simulink library "LIB_TIME"  (Simulink 8.8)
settings: Solver=ode45  StartTime=0.0  StopTime=10.0  RelTol=1e-3  EnableMultiTasking=on
settings Model: Creator=alger  LastModifiedBy=alger

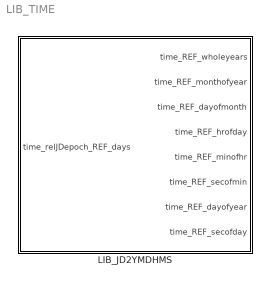
== system LIB_TIME ==
  LIB_JD2YMDHMS : Subsystem  TreatAsAtomicUnit=on

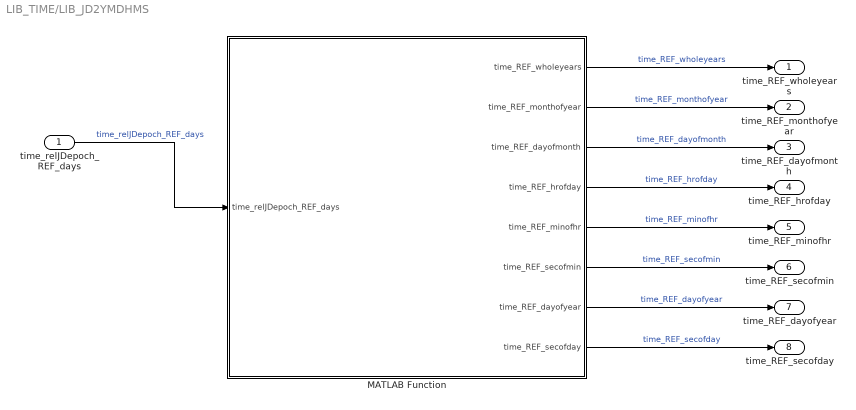
== system LIB_TIME/LIB_JD2YMDHMS ==
  time_relJDepoch_REF_days : Inport
  MATLAB Function : MATLAB Function  TreatAsAtomicUnit=on
  time_REF_wholeyears : Outport
  time_REF_monthofyear : Outport  Port=2
  time_REF_dayofmonth : Outport  Port=3
  time_REF_hrofday : Outport  Port=4
  time_REF_minofhr : Outport  Port=5
  time_REF_secofmin : Outport  Port=6
  time_REF_dayofyear : Outport  Port=7
  time_REF_secofday : Outport  Port=8
  wires:
  MATLAB Function/3(time_REF_dayofmonth) -> time_REF_dayofmonth/1  "time_REF_dayofmonth"
  MATLAB Function/4(time_REF_hrofday) -> time_REF_hrofday/1  "time_REF_hrofday"
  time_relJDepoch_REF_days/1 -> MATLAB Function/1(time_relJDepoch_REF_days)  "time_relJDepoch_REF_days"
  MATLAB Function/1(time_REF_wholeyears) -> time_REF_wholeyears/1  "time_REF_wholeyears"
  MATLAB Function/2(time_REF_monthofyear) -> time_REF_monthofyear/1  "time_REF_monthofyear"
  MATLAB Function/6(time_REF_secofmin) -> time_REF_secofmin/1  "time_REF_secofmin"
  MATLAB Function/8(time_REF_secofday) -> time_REF_secofday/1  "time_REF_secofday"
  MATLAB Function/7(time_REF_dayofyear) -> time_REF_dayofyear/1  "time_REF_dayofyear"
  MATLAB Function/5(time_REF_minofhr) -> time_REF_minofhr/1  "time_REF_minofhr"

== matlab function LIB_JD2YMDHMS/MATLAB Function ==
  data: time_relJDepoch_REF_days input double; time_REF_wholeyears output double; time_REF_monthofyear output double; time_REF_dayofmonth output double; time_REF_hrofday output double; time_REF_minofhr output double; time_REF_secofmin output double; time_REF_dayofyear output double; time_REF_secofday output double
function [...
    time_REF_wholeyears,  ...
    time_REF_monthofyear, ...
    time_REF_dayofmonth,  ...
    time_REF_hrofday,     ...
    time_REF_minofhr,     ...
    time_REF_secofmin,    ...
    time_REF_dayofyear,   ...
    time_REF_secofday ] = call_jd2ymdhms(time_relJDepoch_REF_days)
  %#codegen
  
  [time_REF_wholeyears,...
    time_REF_monthofyear,...
    time_REF_dayofmonth,...
    time_REF_hrofday,...
    time_REF_minofhr,...
    time_REF_secofmin,...
    time_REF_dayofyear,...
    time_REF_secofday ] = jd2ymdhms(time_relJDepoch_REF_days);
end
